simulink model "sim1"  (R2019a)
settings: Solver=FixedStepAuto  StartTime=0.0  StopTime=3  FixedStep=0.001  RelTol=1e-3
libraries: simulink x5
settings Model: Creator=robot  LastModifiedBy=robot
settings OptimizationCC: DefaultParameterBehavior=Inlined  EnhancedBackFolding=on  PassReuseOutputArgsAs=Individual arguments  OptimizeBlockOrder=speed  DifferentSizesBufferReuse=on  OptimizationCustomize=off
settings DebuggingCC: ParameterTunabilityLossMsg=error
settings SFSimCC: MATLABDynamicMemAlloc=off
settings RTWCC: SystemTargetFile=ert.tlc  GenCodeOnly=on  PackageName=PID_C++  TemplateMakefile=ert_default_tmf  GenerateReport=on  IncludeHyperlinkInReport=on  LaunchReport=on  TargetLang=C++  GenerateTraceInfo=on  GenerateTraceReport=on  GenerateTraceReportSl=on  GenerateTraceReportSf=on  GenerateTraceReportEml=on
settings CodeAppCC: ForceParamTrailComments=on  IgnoreCustomStorageClasses=off  OperatorAnnotations=on  SimulinkDataObjDesc=on  SFDataObjDesc=on  InsertBlockDesc=on
settings ERTTargetCC: TargetLangStandard=C++03 (ISO)  GenerateSampleERTMain=on  MultiInstanceERTCode=on  CodeInterfacePackaging=C++ class  InlinedParameterPlacement=NonHierarchical  RootIOFormat=Structure reference  ERTCustomFileTemplate=example_file_process.tlc

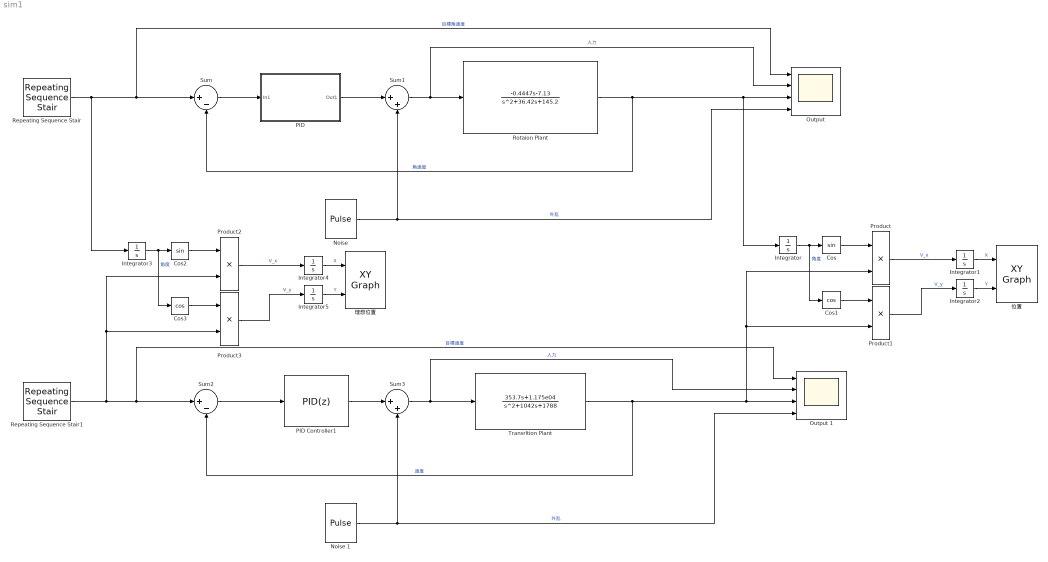
== system sim1 ==
  Cos : Trigonometry
  Cos1 : Trigonometry  Operator=cos
  Cos2 : Trigonometry
  Cos3 : Trigonometry  Operator=cos
  Integrator{,1..5} (6 alike) : Integrator
  "Noise " : DiscretePulseGenerator  PulseType=Time based  Amplitude=0  Period=0.1  PulseWidth=50
  Noise 1 : DiscretePulseGenerator  PulseType=Time based  Amplitude=0  Period=0.1  PulseWidth=50
  "Output " : Scope  NumInputPorts=4
  Output 1 : Scope  NumInputPorts=4
  "PID " : Subsystem  TreatAsAtomicUnit=on
  PID Controller1 : simulink/Continuous/PID Controller  Controller=PID  Form=Parallel  TimeDomain=Discrete-time  SampleTime=0.001  IntegratorMethod=Forward Euler  FilterMethod=Forward Euler  ControllerParametersSource=internal  P=0.73598  I=3.7518  D=0  UseFilter=on  N=100  TunerSelectOption=Transfer Function Based (PID Tuner App)  InitialConditionSource=internal  InitialConditionForIntegrator=0  InitialConditionForFilter=0  DifferentiatorICPrevScaledInput=0  ExternalReset=none  TrackingMode=off  Kt=1  LimitOutput=on  UpperSaturationLimit=1200  LowerSaturationLimit=-1200  LinearizeAsGain=on  AntiWindupMode=none  Kb=1  POutMin=[]  POutMax=[]  IOutMin=[]  IOutMax=[]  DOutMin=[]  DOutMax=[]  NOutMin=[]  NOutMax=[]  SumOutMin=[]  SumOutMax=[]  SaturationOutMin=[]  SaturationOutMax=[]  PParamMin=[]  PParamMax=[]  IParamMin=[]  IParamMax=[]  DParamMin=[]  DParamMax=[]  NParamMin=[]  NParamMax=[]  KbParamMin=[]  KbParamMax=[]  KtParamMin=[]  KtParamMax=[]  KbOutMin=[]  KbOutMax=[]  KtOutMin=[]  KtOutMax=[]  IntegratorOutMin=[]  IntegratorOutMax=[]  FilterOutMin=[]  FilterOutMax=[]  SumI1OutMin=[]  SumI1OutMax=[]  SumI2OutMin=[]  SumI2OutMax=[]  SumI3OutMin=[]  SumI3OutMax=[]  SumI4OutMin=[]  SumI4OutMax=[]  SumDOutMin=[]  SumDOutMax=[]  DifferentiatorOutMin=[]  DifferentiatorOutMax=[]  FilterDiffOutCoefMin=[]  FilterDiffOutCoefMax=[]  ReciprocalOutMin=[]  ReciprocalOutMax=[]  SumDenOutMin=[]  SumDenOutMax=[]  SumNumOutMin=[]  SumNumOutMax=[]  DivideOutMin=[]  DivideOutMax=[]  IntegratorContinuousStateAttributes=''  IntegratorStateMustResolveToSignalObject=off  IntegratorRTWStateStorageClass=Auto  FilterContinuousStateAttributes=''  FilterStateMustResolveToSignalObject=off  FilterRTWStateStorageClass=Auto  ParallelPVariant=InternalParameters  IdealPVariant=Disabled  IVariant=InternalParameters  DVariant=InternalParameters  IntegratorVariant=Discrete  SatVariant=Enabled  AWVariant=Passthrough  PCopyVariant=Disabled  TRVariant=Disabled  FdbkBlocksVariant=Forward  IdealPFdbkVariant=Disabled  SatFdbkVariant=Disabled  DerivativeFilterVariant=ForwardEulerFilter  NVariant=InternalParameters  NCopyVariant=Disabled  FilterICVariant=InternalICsFilter  IntegratorICVariant=InternalICs  ExternalResetVariant=Disabled  TRSumVariant=Passthrough  SumFdbkVariant=Disabled  SumVariant=Sum_PID
  Product{,1..3} (4 alike) : Product
  Repeating Sequence Stair : simulink/Sources/Repeating Sequence Stair  OutValues=[10 15 20].'  tsamp=1  OutMin=[]  OutMax=[]  OutDataTypeStr=double  OutputDataTypeScalingMode=double  OutDataType=fixdt(0,8)  ConRadixGroup=Best Precision: Vector-wise  OutScaling=2^-12
  Repeating Sequence Stair1 : simulink/Sources/Repeating Sequence Stair  OutValues=100  tsamp=1  OutMin=[]  OutMax=[]  OutDataTypeStr=double  OutputDataTypeScalingMode=double  OutDataType=fixdt(0,8)  ConRadixGroup=Best Precision: Vector-wise  OutScaling=2^-12
  Rotaion Plant : TransferFcn  Numerator=[-0.4447 -7.13]  Denominator=[1 36.42 145.2]
  Sum : Sum  Inputs=|+-
  Sum1 : Sum  Inputs=|++
  Sum2 : Sum  Inputs=|+-
  Sum3 : Sum  Inputs=|++
  Transrltion Plant : TransferFcn  Numerator=[353.7 1.175e04]  Denominator=[1 1042 1788]
  "位置 " : simulink/Sinks/XY Graph  xmin=-20  xmax=20  ymin=-20  ymax=20  st=0.001
  理想位置 : simulink/Sinks/XY Graph  xmin=-20  xmax=20  ymin=-20  ymax=20  st=0.001
  wires:
  Sum/1 -> "PID "/1(In1)
  Rotaion Plant/1 -> Sum/2, Integrator/1, "Output "/3  "角速度"
  "PID "/1(Out1) -> Sum1/1
  Sum1/1 -> "Output "/2, Rotaion Plant/1  "入力"
  "Noise "/1 -> "Output "/4, Sum1/2  "外乱"
  Transrltion Plant/1 -> Product/2, Product1/2, Output 1/3, Sum2/2  "速度"
  Sum3/1 -> Output 1/2, Transrltion Plant/1  "入力"
  PID Controller1/1 -> Sum3/1
  Sum2/1 -> PID Controller1/1
  Noise 1/1 -> Output 1/4, Sum3/2  "外乱"
  Cos/1 -> Product/1
  Product/1 -> Integrator1/1  "V_x"
  Cos1/1 -> Product1/1
  Integrator/1 -> Cos1/1, Cos/1  "角度"
  Product1/1 -> Integrator2/1  "V_y"
  Integrator1/1 -> "位置 "/1  "X"
  Integrator2/1 -> "位置 "/2  "Y"
  Repeating Sequence Stair/1 -> Integrator3/1, "Output "/1, Sum/1  "目標角速度"
  Repeating Sequence Stair1/1 -> Product3/2, Product2/2, Output 1/1, Sum2/1  "目標速度"
  Product3/1 -> Integrator5/1  "V_y"
  Integrator5/1 -> 理想位置/2  "Y"
  Cos3/1 -> Product3/1
  Cos2/1 -> Product2/1
  Product2/1 -> Integrator4/1  "V_x"
  Integrator3/1 -> Cos3/1, Cos2/1  "角度"
  Integrator4/1 -> 理想位置/1  "X"

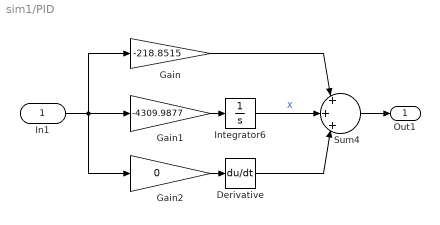
== system sim1/PID  ==
  In1 : Inport
  Derivative : Derivative
  Gain : Gain  Gain=-218.8515
  Gain1 : Gain  Gain=-4309.9877
  Gain2 : Gain  Gain=0
  Integrator6 : Integrator
  Sum4 : Sum  Inputs=|+|+|+|
  Out1 : Outport
  wires:
  Integrator6/1 -> Sum4/2  "X"
  Gain2/1 -> Derivative/1
  Derivative/1 -> Sum4/3
  Gain1/1 -> Integrator6/1
  Gain/1 -> Sum4/1
  Sum4/1 -> Out1/1
  In1/1 -> Gain2/1, Gain/1, Gain1/1
